simulink model "modelo_motor_P3"  (R2021b)
settings: Solver=VariableStepAuto  StartTime=0.0  StopTime=T_end  RelTol=1e-3
values from neighbouring files (symbols this model uses):
  Gz = c2d(G,Tm)    [lanza_P3.m]
  k_nl = 3.6    [lanza_P3.m]
  Tm = 0.01    [lanza_P3.m]
  V_dead = 1    [lanza_P3.m]
  V_sat = 9.5    [lanza_P3.m]
libraries: cstblocks x4, dspsrcs4 x2
settings Model: Creator=jvalls  LastModifiedBy=pasallla
settings SolverCC: AlgebraicLoopSolver=TrustRegion
settings DataIOCC: ReturnWorkspaceOutputs=off
settings OptimizationCC: LifeSpan=inf
settings DebuggingCC: SFMachineParentedDataDiag=warning  ArithmeticOperatorsInVariantConditions=warning
settings SFSimCC: SimUseLocalCustomCode=off  CustomCodeUndefinedFunction=UseInterfaceOnly
settings RTWCC: RTWUseLocalCustomCode=off
settings CodeAppCC: StateflowObjectComments=on

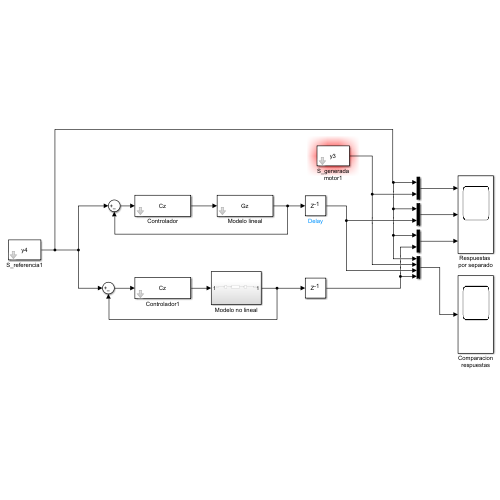
[thumbnail: Simulink's stored preview of the top-level diagram]
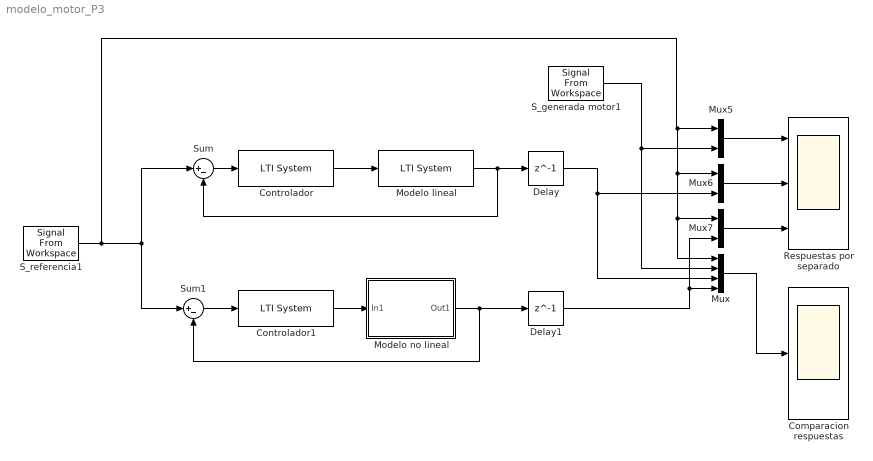
== system modelo_motor_P3 ==
  Comparacion respuestas : Scope
  Controlador : cstblocks/LTI System  sys=Cz  IC=[]
  Controlador1 : cstblocks/LTI System  sys=Cz  IC=[]
  Delay : Delay  DelayLength=1  InitialCondition=0
  Delay1 : Delay  DelayLength=1  InitialCondition=0
  Modelo lineal : cstblocks/LTI System  sys=Gz  IC=[]
  "Modelo no lineal " : Subsystem
  Mux : Mux
  Mux5 : Mux  Inputs=2
  Mux6 : Mux  Inputs=2
  Mux7 : Mux  Inputs=2
  Respuestas por separado : Scope  NumInputPorts=3
  S_generada motor1 : dspsrcs4/Signal From Workspace  X=y3  Ts=Tm  nsamps=1  OutputAfterFinalValue=Setting to zero  ignoreOrWarnInputAndFrameLengths=off  OutputFrames=off
  S_referencia1 : dspsrcs4/Signal From Workspace  X=y4  Ts=Tm  nsamps=1  OutputAfterFinalValue=Setting to zero  ignoreOrWarnInputAndFrameLengths=off  OutputFrames=off
  Sum : Sum  Inputs=|+-
  Sum1 : Sum  Inputs=|+-
  wires:
  S_referencia1/1 -> Mux5/1, Mux6/1, Mux7/1, Mux/1, Sum1/1, Sum/1
  Mux5/1 -> Respuestas por separado/1
  S_generada motor1/1 -> Mux5/2, Mux/2
  Mux/1 -> Comparacion respuestas/1
  Mux7/1 -> Respuestas por separado/3
  Mux6/1 -> Respuestas por separado/2
  Sum/1 -> Controlador/1
  Controlador/1 -> Modelo lineal/1
  Sum1/1 -> Controlador1/1
  Controlador1/1 -> "Modelo no lineal "/1(In1)
  Modelo lineal/1 -> Delay/1, Sum/2
  "Modelo no lineal "/1(Out1) -> Delay1/1, Sum1/2
  Delay/1 -> Mux6/2, Mux/3
  Delay1/1 -> Mux7/2, Mux/4

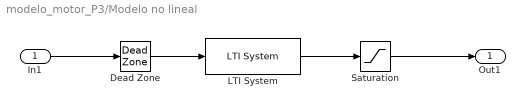
== system modelo_motor_P3/Modelo no lineal  ==
  In1 : Inport
  "Dead Zone " : DeadZone  LowerValue=-V_dead  UpperValue=V_dead
  "LTI System " : cstblocks/LTI System  sys=Gz*k_nl  IC=[]
  "Saturation " : Saturate  UpperLimit=V_sat  LowerLimit=-V_sat
  Out1 : Outport
  wires:
  "Dead Zone "/1 -> "LTI System "/1
  In1/1 -> "Dead Zone "/1
  "Saturation "/1 -> Out1/1
  "LTI System "/1 -> "Saturation "/1
